simulink library "MOTH"  (R2016a)
settings: Solver=ode45  StartTime=0.0  StopTime=10.0  RelTol=1e-3
undefined symbols (not defined in the file): BACKWARD, FORWARD, MOTOR_HIGH, MOTOR_LOW, STOP
libraries: simulink x1
settings Model: Creator=oelkawok  LastModifiedBy=oelkawok
settings DataIOCC: LimitDataPoints=on
settings DebuggingCC: AllowSymbolicDim=off

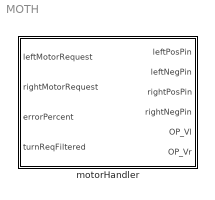
== system MOTH ==
  motorHandler : Subsystem

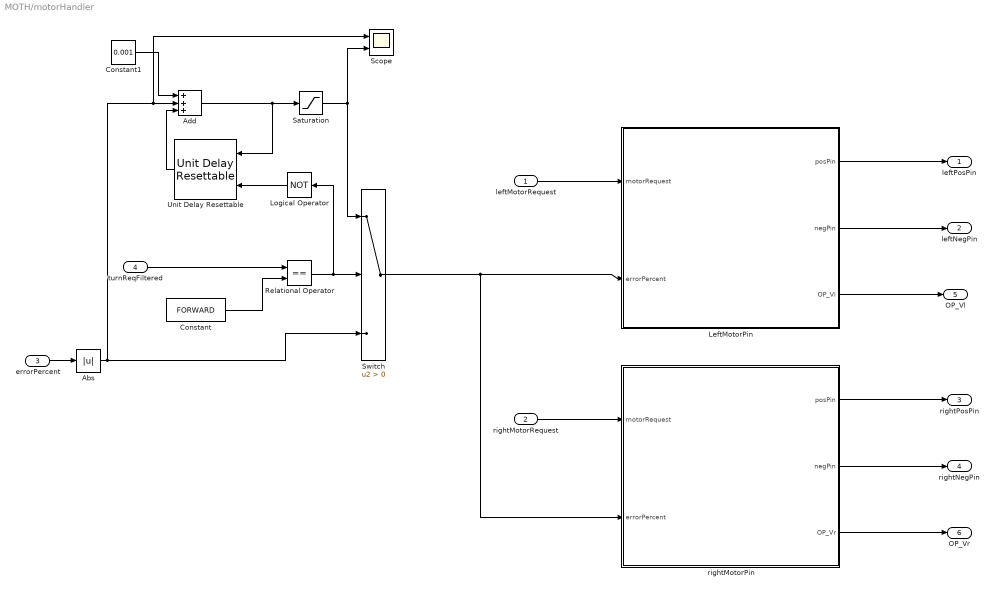
== system MOTH/motorHandler ==
  leftMotorRequest : Inport
  rightMotorRequest : Inport  Port=2
  errorPercent : Inport  Port=3
  turnReqFiltered : Inport  Port=4
  Abs : Abs
  Add : Sum  Inputs=+++
  Constant : Constant  Value=FORWARD
  Constant1 : Constant  Value=0.001
  LeftMotorPin : Subsystem
  Logical Operator : Logic  Operator=NOT  AllPortsSameDT=off  OutDataTypeStr=boolean
  Relational Operator : RelationalOperator  Operator===  OutDataTypeStr=boolean
  Saturation : Saturate  LowerLimit=0
  Scope : Scope  NumInputPorts=2
  Switch : Switch  Criteria=u2 > Threshold
  Unit Delay Resettable : simulink/Additional Math & Discrete/Additional Discrete/Unit Delay Resettable  vinit=0.001  tsamp=-1
  rightMotorPin : Subsystem
  leftPosPin : Outport
  leftNegPin : Outport  Port=2
  rightPosPin : Outport  Port=3
  rightNegPin : Outport  Port=4
  OP_Vl : Outport  Port=5
  OP_Vr : Outport  Port=6
  wires:
  Logical Operator/1 -> Unit Delay Resettable/2
  Constant1/1 -> Add/1
  Relational Operator/1 -> Switch/2, Logical Operator/1
  Saturation/1 -> Scope/2, Switch/1
  Add/1 -> Saturation/1, Unit Delay Resettable/1
  Unit Delay Resettable/1 -> Add/3
  Switch/1 -> LeftMotorPin/2(errorPercent), rightMotorPin/2(errorPercent)
  Abs/1 -> Switch/3, Add/2, Scope/1
  Constant/1 -> Relational Operator/2
  turnReqFiltered/1 -> Relational Operator/1
  errorPercent/1 -> Abs/1
  rightMotorRequest/1 -> rightMotorPin/1(motorRequest)
  rightMotorPin/2(negPin) -> rightNegPin/1
  rightMotorPin/1(posPin) -> rightPosPin/1
  LeftMotorPin/2(negPin) -> leftNegPin/1
  LeftMotorPin/1(posPin) -> leftPosPin/1
  leftMotorRequest/1 -> LeftMotorPin/1(motorRequest)
  LeftMotorPin/3(OP_Vl) -> OP_Vl/1
  rightMotorPin/3(OP_Vr) -> OP_Vr/1

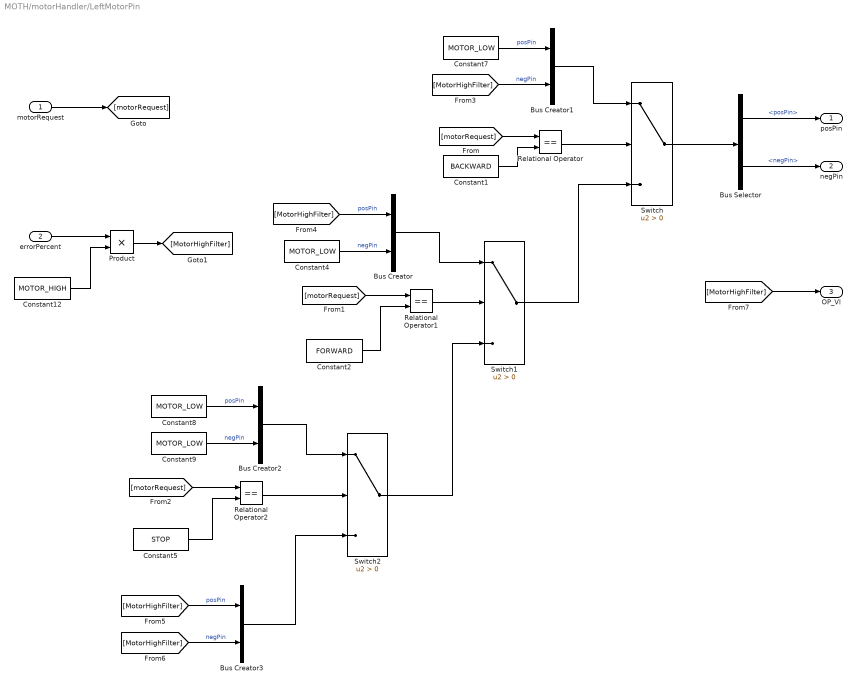
== system MOTH/motorHandler/LeftMotorPin ==
  motorRequest : Inport
  errorPercent : Inport  Port=2
  Bus Creator{,1..3} (4 alike) : BusCreator  Inputs=2
  Bus Selector : BusSelector  OutputSignals=posPin,negPin
  Constant1 : Constant  Value=BACKWARD
  Constant12 : Constant  Value=MOTOR_HIGH
  Constant2 : Constant  Value=FORWARD
  Constant{4,7..9} (4 alike) : Constant  Value=MOTOR_LOW
  Constant5 : Constant  Value=STOP
  Product : Product
  Relational Operator : RelationalOperator  Operator===  OutDataTypeStr=boolean
  Relational Operator1 : RelationalOperator  Operator===  OutDataTypeStr=boolean
  Relational Operator2 : RelationalOperator  Operator===  OutDataTypeStr=boolean
  Switch : Switch  Criteria=u2 > Threshold
  Switch1 : Switch  Criteria=u2 > Threshold
  Switch2 : Switch  Criteria=u2 > Threshold
  posPin : Outport
  negPin : Outport  Port=2
  OP_Vl : Outport  Port=3
  wires:
  Bus Selector/2 -> negPin/1  "<negPin>"
  Bus Selector/1 -> posPin/1  "<posPin>"
  Switch/1 -> Bus Selector/1
  [motorRequest] -> Relational Operator1/1
  [motorRequest] -> Relational Operator/1
  motorRequest/1 -> [motorRequest]
  Bus Creator3/1 -> Switch2/3
  Switch2/1 -> Switch1/3
  [MotorHighFilter] -> Bus Creator3/1  "posPin"
  Constant9/1 -> Bus Creator2/2  "negPin"
  Relational Operator2/1 -> Switch2/2
  [MotorHighFilter] -> Bus Creator3/2  "negPin"
  [motorRequest] -> Relational Operator2/1
  Bus Creator1/1 -> Switch/1
  Bus Creator2/1 -> Switch2/1
  Bus Creator/1 -> Switch1/1
  Constant8/1 -> Bus Creator2/1  "posPin"
  Switch1/1 -> Switch/3
  Constant7/1 -> Bus Creator1/1  "posPin"
  Constant5/1 -> Relational Operator2/2
  Constant2/1 -> Relational Operator1/2
  Relational Operator/1 -> Switch/2
  Constant1/1 -> Relational Operator/2
  [MotorHighFilter] -> Bus Creator1/2  "negPin"
  [MotorHighFilter] -> Bus Creator/1  "posPin"
  Constant4/1 -> Bus Creator/2  "negPin"
  Relational Operator1/1 -> Switch1/2
  errorPercent/1 -> Product/1
  Constant12/1 -> Product/2
  Product/1 -> [MotorHighFilter]
  [MotorHighFilter] -> OP_Vl/1

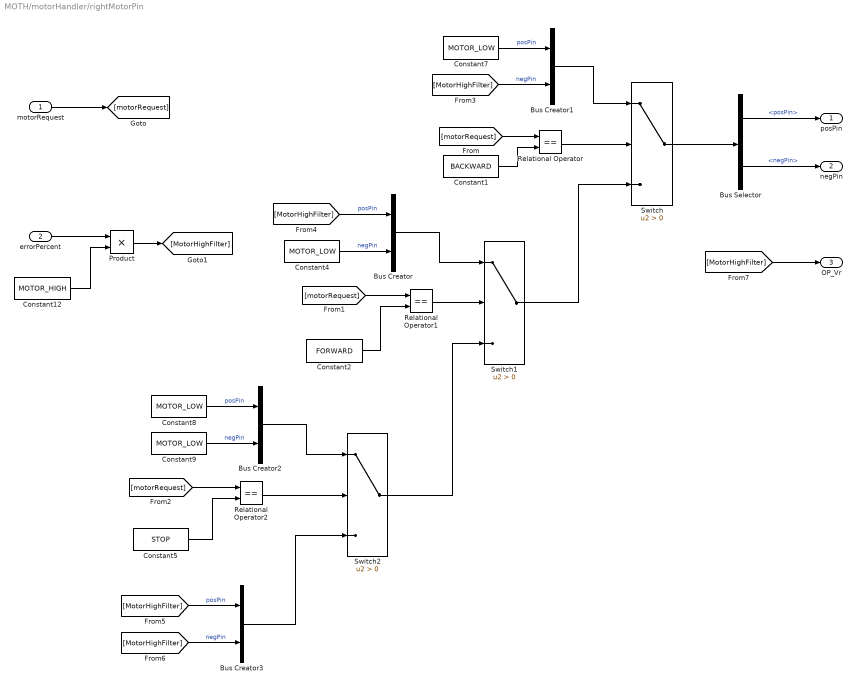
== system MOTH/motorHandler/rightMotorPin ==
  motorRequest : Inport
  errorPercent : Inport  Port=2
  Bus Creator{,1..3} (4 alike) : BusCreator  Inputs=2
  Bus Selector : BusSelector  OutputSignals=posPin,negPin
  Constant1 : Constant  Value=BACKWARD
  Constant12 : Constant  Value=MOTOR_HIGH
  Constant2 : Constant  Value=FORWARD
  Constant{4,7..9} (4 alike) : Constant  Value=MOTOR_LOW
  Constant5 : Constant  Value=STOP
  Product : Product
  Relational Operator : RelationalOperator  Operator===  OutDataTypeStr=boolean
  Relational Operator1 : RelationalOperator  Operator===  OutDataTypeStr=boolean
  Relational Operator2 : RelationalOperator  Operator===  OutDataTypeStr=boolean
  Switch : Switch  Criteria=u2 > Threshold
  Switch1 : Switch  Criteria=u2 > Threshold
  Switch2 : Switch  Criteria=u2 > Threshold
  posPin : Outport
  negPin : Outport  Port=2
  OP_Vr : Outport  Port=3
  wires:
  Product/1 -> [MotorHighFilter]
  Constant12/1 -> Product/2
  errorPercent/1 -> Product/1
  Relational Operator1/1 -> Switch1/2
  Constant4/1 -> Bus Creator/2  "negPin"
  [MotorHighFilter] -> Bus Creator/1  "posPin"
  [MotorHighFilter] -> Bus Creator1/2  "negPin"
  Constant1/1 -> Relational Operator/2
  Relational Operator/1 -> Switch/2
  Constant2/1 -> Relational Operator1/2
  Constant5/1 -> Relational Operator2/2
  Constant7/1 -> Bus Creator1/1  "posPin"
  Switch1/1 -> Switch/3
  Constant8/1 -> Bus Creator2/1  "posPin"
  Bus Creator/1 -> Switch1/1
  Bus Creator2/1 -> Switch2/1
  Bus Creator1/1 -> Switch/1
  [motorRequest] -> Relational Operator2/1
  [MotorHighFilter] -> Bus Creator3/2  "negPin"
  Relational Operator2/1 -> Switch2/2
  Constant9/1 -> Bus Creator2/2  "negPin"
  [MotorHighFilter] -> Bus Creator3/1  "posPin"
  Switch2/1 -> Switch1/3
  Bus Creator3/1 -> Switch2/3
  motorRequest/1 -> [motorRequest]
  [motorRequest] -> Relational Operator/1
  [motorRequest] -> Relational Operator1/1
  Switch/1 -> Bus Selector/1
  Bus Selector/1 -> posPin/1  "<posPin>"
  Bus Selector/2 -> negPin/1  "<negPin>"
  [MotorHighFilter] -> OP_Vr/1
